simulink model "optimizeTest1Sim"  (R2021a)
settings: Solver=VariableStepDiscrete  StartTime=0.0  StopTime=inf  MaxStep=tStep  RelTol=1e-3
values from neighbouring files (symbols this model uses):
  motor1 = Motor('P8175(SL).ric')    [optimizeTest1.m]    (also in optimize_handler.m)
  stage2IgnitionAlt = value    [optS2ignitionAlt.m]    (also in optimizeTest1.m = bestIgnitionAlt; optimizer.m = points(counter, 2))
libraries: eeGeneralControl x2, simulink x1
settings Model: Creator=e406594  LastModifiedBy=ctvnu
settings SolverCC: AlgebraicLoopSolver=TrustRegion
settings DebuggingCC: SFMachineParentedDataDiag=warning

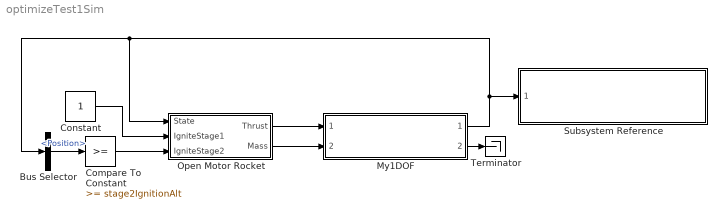
== system optimizeTest1Sim ==
  Bus Selector : BusSelector  OutputSignals=Pose.Position
  Compare To Constant : simulink/Logic and Bit Operations/Compare To Constant  relop=>=  const=stage2IgnitionAlt  OutDataTypeStr=boolean
  Constant : Constant
  My1DOF : Subsystem  ReferencedSubsystem=My1DOF
  Open Motor Rocket : Subsystem  VariantControl=Choice  mask{motor2=motor1, mass2=25, printI2=off, printT2=off, motor1=motor1, mass1=20, printI1=off, printT1=off}
      mask prompts: motor2 "Stage 2 Motor"; mass2 "Stage 2 Dry Mass"; printI2 "Print Impulse"; printT2 "Print Table"; motor1 "Stage 1 Motor"; mass1 "Stage 1 Dry Mass"; printI1 "Print Impulse"; printT1 "Print Table"
      mask DialogControl ParameterGroupVar Prompt: Stage 2 (Upper) Parameters
      mask DialogControl ParameterGroupVar_copy Prompt: Stage 1 (Lower) Parameters
  Subsystem Reference : Subsystem  ReferencedSubsystem=Velocity_based_Simulation_Stop  simTermVel=-10  enableSimTerm=on
  Terminator : Terminator
  wires:
  Open Motor Rocket/1(Thrust) -> My1DOF/1
  Open Motor Rocket/2(Mass) -> My1DOF/2
  Compare To Constant/1 -> Open Motor Rocket/3(IgniteStage2)
  Bus Selector/1 -> Compare To Constant/1  "<Position>"
  Constant/1 -> Open Motor Rocket/2(IgniteStage1)
  My1DOF/1 -> Bus Selector/1, Open Motor Rocket/1(State), Subsystem Reference/1
  My1DOF/2 -> Terminator/1

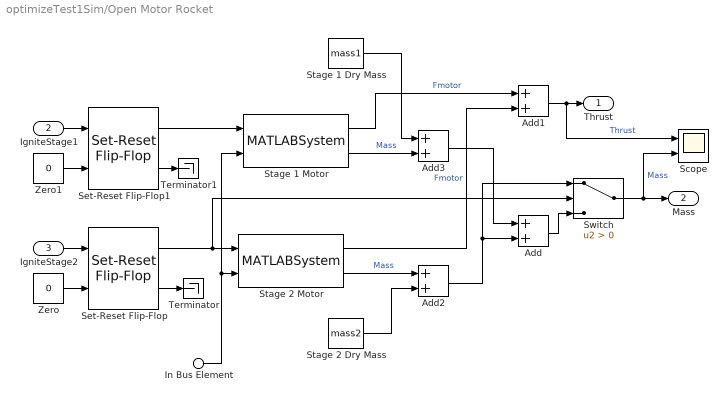
== system optimizeTest1Sim/Open Motor Rocket ==
  In Bus Element : Inport  PortName=State  Element=Atmos.P
  IgniteStage1 : Inport  Port=2
  IgniteStage2 : Inport  Port=3
  Add{,1..3} (4 alike) : Sum
  Scope : Scope  NumInputPorts=2
  Set-Reset Flip-Flop : eeGeneralControl/Set-Reset Flip-Flop  LabelModeActiveChoice=Discrete  UndefState=Set  Q0=0  Ts=-1
      settings: SourceProductBaseCode=PS
  Set-Reset Flip-Flop1 : eeGeneralControl/Set-Reset Flip-Flop  LabelModeActiveChoice=Discrete  UndefState=Set  Q0=0  Ts=-1
      settings: SourceProductBaseCode=PS
  Stage 1 Dry Mass : Constant  Value=mass1
  Stage 1 Motor : MATLABSystem  System=MotorSystem  tStep=tStep  motorStruct=motor1.getStruct()  printImpulse=printI1  printTable=printT1  SimulateUsing=Code generation
      mask Type: MotorSystem
      mask Display:
      | disp('MotorSystem');
      | port_label('input',1,'start');
      | port_label('input',2,'ambPressure');
      | port_label('output',1,'thrust');
      | port_label('output',2,'mass');
  Stage 2 Dry Mass : Constant  Value=mass2
  Stage 2 Motor : MATLABSystem  System=MotorSystem  tStep=tStep  motorStruct=motor2.getStruct()  printImpulse=printI2  printTable=printT2  SimulateUsing=Code generation
      mask Type: MotorSystem
      mask Display:
      | disp('MotorSystem');
      | port_label('input',1,'start');
      | port_label('input',2,'ambPressure');
      | port_label('output',1,'thrust');
      | port_label('output',2,'mass');
  Switch : Switch  Criteria=u2 > Threshold
  Terminator : Terminator
  Terminator1 : Terminator
  Zero : Constant  Value=0  OutDataTypeStr=Inherit: Inherit via back propagation
  Zero1 : Constant  Value=0  OutDataTypeStr=Inherit: Inherit via back propagation
  Thrust : Outport
  Mass : Outport  Port=2
  wires:
  Set-Reset Flip-Flop1/1 -> Stage 1 Motor/1
  Switch/1 -> Scope/2, Mass/1  "Mass"
  Add1/1 -> Scope/1, Thrust/1  "Thrust"
  Stage 2 Motor/1 -> Add1/2  "Fmotor"
  Stage 1 Motor/1 -> Add1/1  "Fmotor"
  Set-Reset Flip-Flop/1 -> Switch/2, Stage 2 Motor/1
  IgniteStage2/1 -> Set-Reset Flip-Flop/1
  Zero/1 -> Set-Reset Flip-Flop/2
  Add/1 -> Switch/3
  Set-Reset Flip-Flop/2 -> Terminator/1
  Zero1/1 -> Set-Reset Flip-Flop1/2
  IgniteStage1/1 -> Set-Reset Flip-Flop1/1
  Set-Reset Flip-Flop1/2 -> Terminator1/1
  In Bus Element/1 -> Stage 1 Motor/2, Stage 2 Motor/2
  Stage 1 Dry Mass/1 -> Add3/1
  Stage 2 Motor/2 -> Add2/1  "Mass"
  Stage 1 Motor/2 -> Add3/2  "Mass"
  Stage 2 Dry Mass/1 -> Add2/2
  Add2/1 -> Switch/1, Add/2
  Add3/1 -> Add/1
